simulink model "fenglixitongmoxing"  (R2014a)
settings: Solver=ode45  StartTime=0.0  StopTime=10.0  RelTol=1e-3
libraries: simulink x1
settings Model: Creator=hsinwang  LastModifiedBy=hsinwang

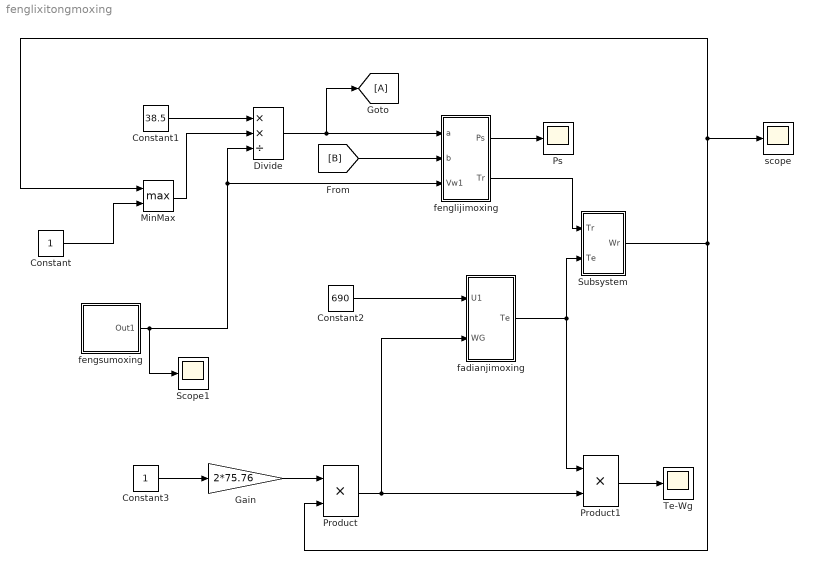
== system fenglixitongmoxing ==
  Constant : Constant
  Constant1 : Constant  Value=38.5
  Constant2 : Constant  Value=690
  Constant3 : Constant
  Divide : Product  Inputs=**/
  Gain : Gain  Gain=2*75.76
  MinMax : MinMax  Function=max  Inputs=2
  Product : Product
  Product1 : Product
  "Ps " : Scope
  Scope1 : Scope
  Subsystem : Subsystem
  "Te-Wg " : Scope
      settings: SaveName=ScopeData2
  "fadianjimoxing " : Subsystem
  "fenglijimoxing " : Subsystem
  fengsumoxing : Subsystem
  "scope " : Scope
      settings: SaveName=ScopeData3
  wires:
  "fenglijimoxing "/2(" Tr ") -> Subsystem/1(Tr)
  "fadianjimoxing "/1(Te) -> Product1/1, Subsystem/2(Te)
  fengsumoxing/1(Out1) -> Divide/3, "fenglijimoxing "/3(Vw1), Scope1/1
  Constant/1 -> MinMax/2
  MinMax/1 -> Divide/2
  Constant1/1 -> Divide/1
  Divide/1 -> [A], "fenglijimoxing "/1("a ")
  [B] -> "fenglijimoxing "/2(b)
  "fenglijimoxing "/1("Ps ") -> "Ps "/1
  Constant2/1 -> "fadianjimoxing "/1(U1)
  Constant3/1 -> Gain/1
  Gain/1 -> Product/1
  Product/1 -> "fadianjimoxing "/2(WG), Product1/2
  Product1/1 -> "Te-Wg "/1
  Subsystem/1(Wr) -> "scope "/1, MinMax/1, Product/2

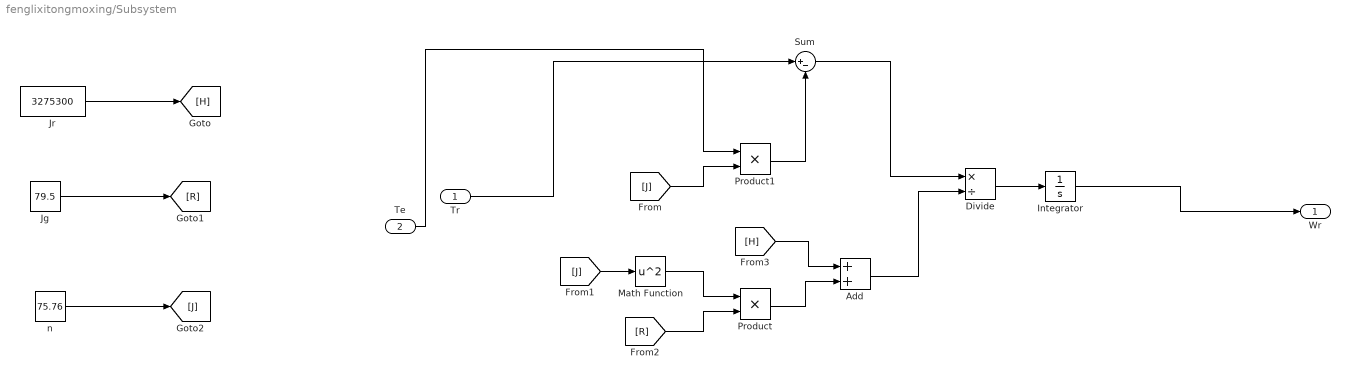
== system fenglixitongmoxing/Subsystem ==
  Tr : Inport
  Te : Inport  Port=2
  Add : Sum
  Divide : Product  Inputs=*/
  Integrator : Integrator
  "Jg " : Constant  Value=79.5
  "Jr " : Constant  Value=3275300
  Math Function : Math  Operator=square  SaturateOnIntegerOverflow=on
  Product : Product
  Product1 : Product
  Sum : Sum  Inputs=|+-
  n : Constant  Value=75.76
  Wr : Outport
  wires:
  Product1/1 -> Sum/2
  [H] -> Add/1
  Sum/1 -> Divide/1
  n/1 -> [J]
  [J] -> Product1/2
  Add/1 -> Divide/2
  Divide/1 -> Integrator/1
  Math Function/1 -> Product/1
  Tr/1 -> Sum/1
  "Jg "/1 -> [R]
  [J] -> Math Function/1
  Integrator/1 -> Wr/1
  "Jr "/1 -> [H]
  Product/1 -> Add/2
  [R] -> Product/2
  Te/1 -> Product1/1

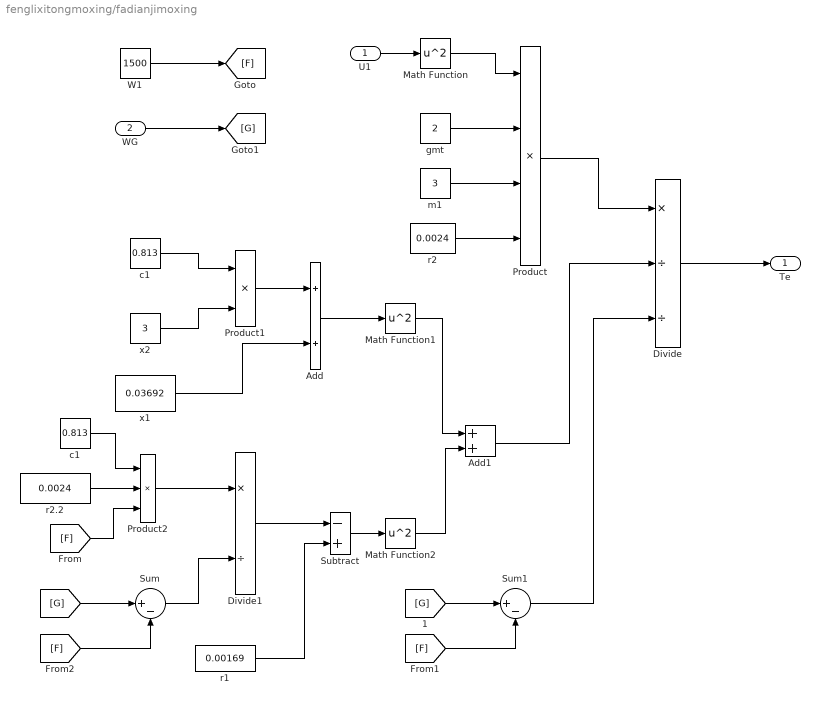
== system fenglixitongmoxing/fadianjimoxing  ==
  U1 : Inport
  WG : Inport  Port=2
  Add : Sum
  Add1 : Sum
  Divide : Product  Inputs=*//
  Divide1 : Product  Inputs=*/
  Math Function : Math  Operator=square  SaturateOnIntegerOverflow=on
  Math Function1 : Math  Operator=square  SaturateOnIntegerOverflow=on
  Math Function2 : Math  Operator=square  SaturateOnIntegerOverflow=on
  Product : Product  Inputs=4
  Product1 : Product
  Product2 : Product  Inputs=3
  Subtract : Sum  Inputs=-+
  Sum : Sum  Inputs=|+-
  Sum1 : Sum  Inputs=|+-
  W1 : Constant  Value=1500
  c1 : Constant  Value=0.813
  "c1 " : Constant  Value=0.813
  gmt : Constant  Value=2
  m1 : Constant  Value=3
  r1 : Constant  Value=0.00169
  r2 : Constant  Value=0.0024
  r2.2 : Constant  Value=0.0024
  "x1 " : Constant  Value=0.03692
  x2 : Constant  Value=3
  Te : Outport
  wires:
  Product1/1 -> Add/1
  Sum/1 -> Divide1/2
  U1/1 -> Math Function/1
  Add/1 -> Math Function1/1
  WG/1 -> [G]
  x2/1 -> Product1/2
  Divide/1 -> Te/1
  "c1 "/1 -> Product1/1
  Product/1 -> Divide/1
  W1/1 -> [F]
  Subtract/1 -> Math Function2/1
  Add1/1 -> Divide/2
  Product2/1 -> Divide1/1
  r2.2/1 -> Product2/2
  r1/1 -> Subtract/2
  [F] -> Sum/2
  Divide1/1 -> Subtract/1
  [G] -> Sum/1
  [F] -> Product2/3
  c1/1 -> Product2/1
  Sum1/1 -> Divide/3
  [G] -> Sum1/1
  [F] -> Sum1/2
  Math Function2/1 -> Add1/2
  Math Function1/1 -> Add1/1
  gmt/1 -> Product/2
  "x1 "/1 -> Add/2
  m1/1 -> Product/3
  Math Function/1 -> Product/1
  r2/1 -> Product/4

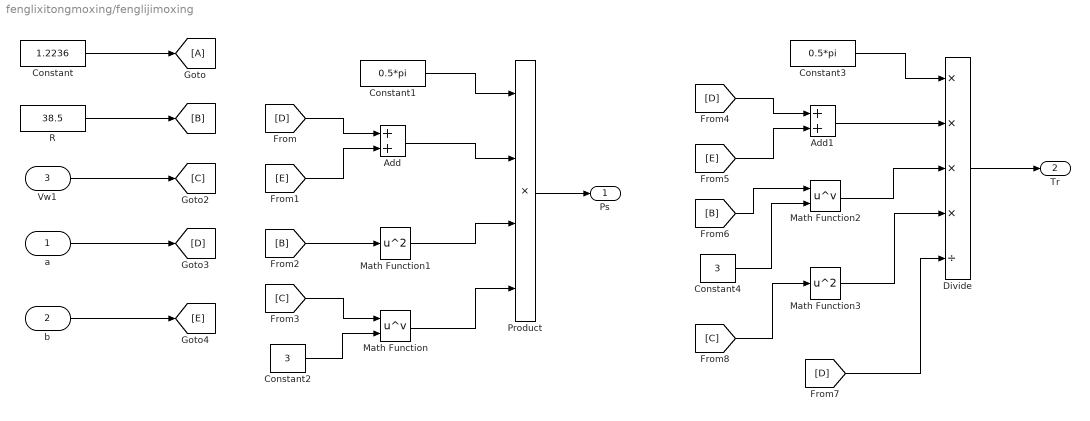
== system fenglixitongmoxing/fenglijimoxing  ==
  "a " : Inport
  b : Inport  Port=2
  Vw1 : Inport  Port=3
  Add : Sum
  Add1 : Sum
  Constant : Constant  Value=1.2236
  Constant1 : Constant  Value=0.5*pi
  Constant2 : Constant  Value=3
  Constant3 : Constant  Value=0.5*pi
  Constant4 : Constant  Value=3
  Divide : Product  Inputs=****/
  Math Function : Math  Operator=pow  SaturateOnIntegerOverflow=on
  Math Function1 : Math  Operator=square  SaturateOnIntegerOverflow=on
  Math Function2 : Math  Operator=pow  SaturateOnIntegerOverflow=on
  Math Function3 : Math  Operator=square  SaturateOnIntegerOverflow=on
  Product : Product  Inputs=4
  R : Constant  Value=38.5
  "Ps " : Outport
  " Tr " : Outport  Port=2
  wires:
  Constant1/1 -> Product/1
  [B] -> Math Function1/1
  Constant2/1 -> Math Function/2
  [C] -> Math Function/1
  "a "/1 -> [D]
  R/1 -> [B]
  b/1 -> [E]
  Vw1/1 -> [C]
  Constant/1 -> [A]
  Add1/1 -> Divide/2
  Divide/1 -> " Tr "/1
  Constant3/1 -> Divide/1
  [E] -> Add1/2
  Math Function/1 -> Product/4
  [E] -> Add/2
  Constant4/1 -> Math Function2/2
  [D] -> Add1/1
  [B] -> Math Function2/1
  Math Function3/1 -> Divide/4
  [D] -> Divide/5
  [D] -> Add/1
  Add/1 -> Product/2
  [C] -> Math Function3/1
  Product/1 -> "Ps "/1
  Math Function1/1 -> Product/3
  Math Function2/1 -> Divide/3

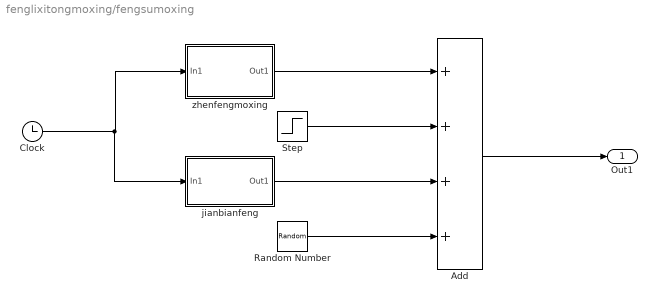
== system fenglixitongmoxing/fengsumoxing ==
  Add : Sum  Inputs=++++
  Clock : Clock
  Random Number : RandomNumber  SampleTime=0.1
  Step : Step  SampleTime=0
  jianbianfeng : Subsystem
  "zhenfengmoxing " : Subsystem
  Out1 : Outport
  wires:
  Clock/1 -> "zhenfengmoxing "/1(In1), jianbianfeng/1(In1)
  "zhenfengmoxing "/1(Out1) -> Add/1
  Step/1 -> Add/2
  Add/1 -> Out1/1
  Random Number/1 -> Add/4
  jianbianfeng/1(Out1) -> Add/3

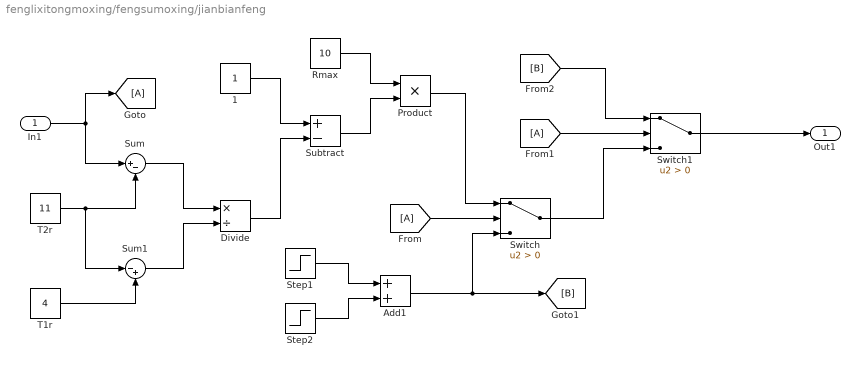
== system fenglixitongmoxing/fengsumoxing/jianbianfeng ==
  In1 : Inport
  1 : Constant
  Add1 : Sum
  Divide : Product  Inputs=*/
  Product : Product
  "Rmax " : Constant  Value=10
  Step1 : Step  SampleTime=0
  Step2 : Step  SampleTime=0
  Subtract : Sum  Inputs=+-
  Sum : Sum  Inputs=|+-
  Sum1 : Sum  Inputs=|-+
  Switch : Switch  Criteria=u2 > Threshold
  Switch1 : Switch  Criteria=u2 > Threshold
  "T1r " : Constant  Value=4
  "T2r " : Constant  Value=11
  Out1 : Outport
  wires:
  In1/1 -> [A], Sum/1
  Switch/1 -> Switch1/3
  Subtract/1 -> Product/2
  "T2r "/1 -> Sum/2, Sum1/1
  "Rmax "/1 -> Product/1
  "T1r "/1 -> Sum1/2
  [A] -> Switch/2
  [B] -> Switch1/1
  Sum1/1 -> Divide/2
  Add1/1 -> [B], Switch/3
  Divide/1 -> Subtract/2
  Switch1/1 -> Out1/1
  Sum/1 -> Divide/1
  Product/1 -> Switch/1
  1/1 -> Subtract/1
  [A] -> Switch1/2
  Step1/1 -> Add1/1
  Step2/1 -> Add1/2

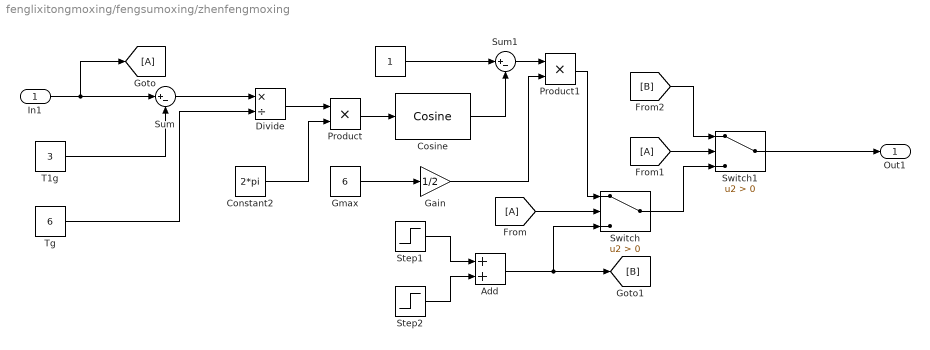
== system fenglixitongmoxing/fengsumoxing/zhenfengmoxing  ==
  In1 : Inport
  " Gmax " : Constant  Value=6
  " " : Constant
  Add : Sum
  Constant2 : Constant  Value=2*pi
  Cosine : simulink/Lookup Tables/Cosine  Formula=cos(2*pi*u)  NumDataPoints=(2^5)+1  OutputWordLength=16  InternalRulePriority=Speed
  Divide : Product  Inputs=*/
  Gain : Gain  Gain=1/2
  Product : Product
  Product1 : Product
  Step1 : Step  SampleTime=0
  Step2 : Step  SampleTime=0
  Sum : Sum  Inputs=|+-
  Sum1 : Sum  Inputs=|+-
  Switch : Switch  Criteria=u2 > Threshold
  Switch1 : Switch  Criteria=u2 > Threshold
  "T1g " : Constant  Value=3
  "Tg " : Constant  Value=6
  Out1 : Outport
  wires:
  [B] -> Switch1/1
  [A] -> Switch1/2
  [A] -> Switch/2
  Add/1 -> Switch/3, [B]
  Switch1/1 -> Out1/1
  Step2/1 -> Add/2
  " "/1 -> Sum1/1
  Step1/1 -> Add/1
  " Gmax "/1 -> Gain/1
  Switch/1 -> Switch1/3
  Gain/1 -> Product1/2
  Sum1/1 -> Product1/1
  Product1/1 -> Switch/1
  Cosine/1 -> Sum1/2
  "Tg "/1 -> Divide/2
  In1/1 -> [A], Sum/1
  "T1g "/1 -> Sum/2
  Sum/1 -> Divide/1
  Constant2/1 -> Product/2
  Divide/1 -> Product/1
  Product/1 -> Cosine/1
